simulink library "csu_rng_range_model_lib"  (R2015b)
settings: Solver=ode45  SolverMode=SingleTasking  StartTime=0.0  StopTime=10.0  RelTol=1e-3
values from neighbouring files (symbols this model uses):
  ldr_null_meas = -100    [csc_ldr_flir_lidar_init.m]
  ldr_use_meme_flag = 0    [csc_ldr_flir_lidar_init.m]
undefined symbols (not defined in the file or in its folder): ini_tgt_landing_mcmf_pos, ldr_100m_percent_error, ldr_100m_range_max, ldr_100m_range_min, ldr_2k_percent_error, ldr_2k_range_max, ldr_2k_range_min, ldr_lander_dcm, ldr_position_in_lander, ldr_rate_counter
libraries: util_quat_lib x9, simulink x6, util_common_lib x6, util_info_lib x3, util_frame_rotation_lib x2, util_geodesy_lib x2
settings Model: Creator=eleanor  LastModifiedBy=Mark Agbayani
settings DataIOCC: SaveFormat=Array  SignalLoggingSaveFormat=ModelDataLogs
settings OptimizationCC: BlockReduction=off  BooleanDataType=off  ExpressionDepthLimit=2147483647
settings DebuggingCC: SaveWithParameterizedLinksMsg=none  UnderspecifiedInitializationDetection=Classic  MergeDetectMultiDrivingBlocksExec=none  SignalResolutionControl=TryResolveAllWithWarning  FcnCallInpInsideContextMsg=EnableAllAsWarning  StateNameClashWarn=warning  StrictBusMsg=Warning
settings HardwareCC: ProdBitPerPointer=32  ProdLargestAtomicFloat=None  ProdIntDivRoundTo=Undefined  ProdEndianess=Unspecified  ProdWordSize=32  ProdHWDeviceType=32-bit Generic  TargetUnknown=on
settings GRTTargetCC: GeneratePreprocessorConditionals=Disable all  CombineOutputUpdateFcns=off  GRTInterface=on
settings ConfigComp: CovModelRefEnable=Off  CovSFcnEnable=off

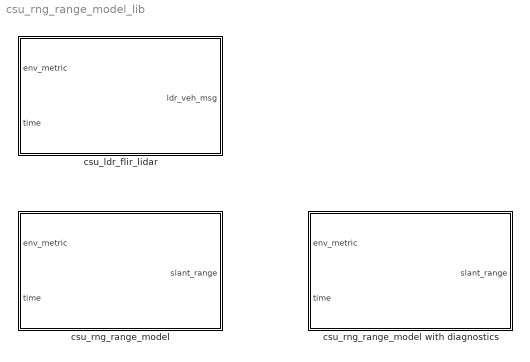
== system csu_rng_range_model_lib ==
  csu_ldr_flir_lidar : Subsystem  SystemSampleTime=0.1
  csu_rng_range_model : Subsystem  SystemSampleTime=0.1  mask{position_in_lander=ldr_position_in_lander, lander_dcm=ldr_lander_dcm}
      mask prompts: position_in_lander "LIDAR Position in Body Frame (meters)"; lander_dcm "LIDAR Attitude wrt Body Frame (DCM)"
  csu_rng_range_model with diagnostics : Subsystem  AncestorBlock=csu_rng_range_model_lib/csu_rng_range_model  SystemSampleTime=0.1  mask{position_in_lander=ldr_position_in_lander, lander_dcm=ldr_lander_dcm}
      mask prompts: position_in_lander "LIDAR Position in Body Frame (meters)"; lander_dcm "LIDAR Attitude wrt Body Frame (DCM)"

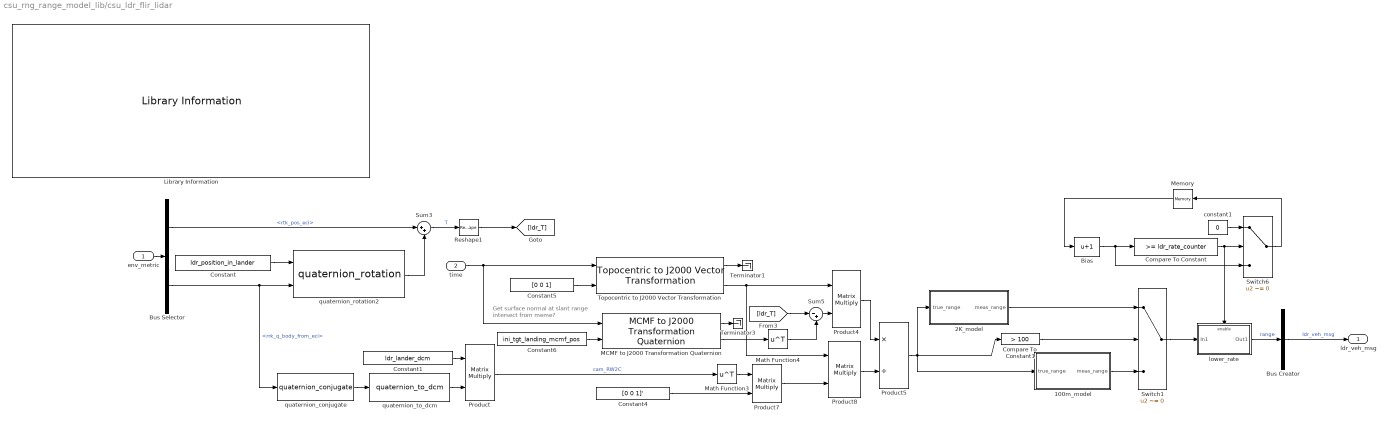
== system csu_rng_range_model_lib/csu_ldr_flir_lidar ==
  note: Get surface normal at slant range
      | intersect from meme?
  env_metric : Inport
  time : Inport  Port=2
  100m_model : Subsystem  TreatAsAtomicUnit=on
  2K_model : Subsystem  TreatAsAtomicUnit=on
  Bias : Bias  Bias=1
  Bus Creator : BusCreator  Inputs=1  OutDataTypeStr=Bus: ldr_veh_msg  NonVirtualBus=on
  Bus Selector : BusSelector  OutputSignals=lander_state_bus.rtk_pos_eci,lander_state_bus.rrk_q_body_from_eci
  Compare To Constant : simulink/Logic and Bit Operations/Compare To Constant  relop=>=  const=ldr_rate_counter  OutDataTypeStr=uint8
  Compare To Constant1 : simulink/Logic and Bit Operations/Compare To Constant  relop=>  const=100  OutDataTypeStr=uint8
  Constant : Constant  Value=ldr_position_in_lander
  Constant1 : Constant  Value=ldr_lander_dcm
  Constant4 : Constant  Value=[0 0 1]'  VectorParams1D=off
  Constant5 : Constant  Value=[0 0 1]  VectorParams1D=off
  Constant6 : Constant  Value=ini_tgt_landing_mcmf_pos  VectorParams1D=off
  Library Information : util_info_lib/Library Information  owner='NONE'
  MCMF to J2000 Transformation Quaternion : util_frame_rotation_lib/MCMF to J2000  Transformation Quaternion
  Math Function3 : Math  Operator=transpose  SaturateOnIntegerOverflow=on
  Math Function4 : Math  Operator=transpose  SaturateOnIntegerOverflow=on
  Memory : Memory  X0=ldr_rate_counter-1  InheritSampleTime=on
  Product{,4,7..8} (4 alike) : Product  Multiplication=Matrix(*)  RndMeth=Zero
  Product5 : Product  Inputs=*/  RndMeth=Zero
  Reshape1 : Reshape  OutputDimensionality=Column vector (2-D)
  Sum3 : Sum  Inputs=|++
  Sum5 : Sum  Inputs=|-+
  Switch1 : Switch  Criteria=u2 ~= 0  InputSameDT=on
  Switch6 : Switch  Criteria=u2 ~= 0  InputSameDT=on
  Terminator1 : Terminator
  Terminator3 : Terminator
  "Topocentric to J2000 Vector Transformation " : util_frame_rotation_lib/Topocentric to J2000 Vector Transformation   SystemSampleTime=-1
  constant1 : Constant  Value=0
  lower_rate : Subsystem  TreatAsAtomicUnit=on
  quaternion_conjugate : util_quat_lib/quaternion_conjugate  SystemSampleTime=-1
  quaternion_rotation2 : util_quat_lib/quaternion_rotation  SystemSampleTime=-1
  quaternion_to_dcm : util_quat_lib/quaternion_to_dcm  SystemSampleTime=-1
  ldr_veh_msg : Outport
  wires:
  quaternion_conjugate/1 -> quaternion_to_dcm/1
  2K_model/1(meas_range) -> Switch1/1
  100m_model/1(meas_range) -> Switch1/3
  Compare To Constant1/1 -> Switch1/2
  Product5/1 -> Compare To Constant1/1, 2K_model/1(true_range), 100m_model/1(true_range)
  Constant4/1 -> Product7/2
  "Topocentric to J2000 Vector Transformation "/1 -> Terminator1/1
  "Topocentric to J2000 Vector Transformation "/2 -> Product8/1, Product4/1
  time/1 -> MCMF to J2000 Transformation Quaternion/1, "Topocentric to J2000 Vector Transformation "/1
  Constant6/1 -> MCMF to J2000 Transformation Quaternion/2
  Constant5/1 -> "Topocentric to J2000 Vector Transformation "/2
  Constant/1 -> quaternion_rotation2/1
  quaternion_rotation2/1 -> Sum3/2
  Constant1/1 -> Product/1
  quaternion_to_dcm/1 -> Product/2
  Math Function4/1 -> Sum5/2
  MCMF to J2000 Transformation Quaternion/1 -> Terminator3/1
  MCMF to J2000 Transformation Quaternion/2 -> Math Function4/1
  Sum5/1 -> Product4/2
  [ldr_T] -> Sum5/1
  Math Function3/1 -> Product7/1
  Reshape1/1 -> [ldr_T]
  Product7/1 -> Product8/2
  env_metric/1 -> Bus Selector/1
  Bus Selector/1 -> Sum3/1  "<rtk_pos_eci>"
  Bus Selector/2 -> quaternion_conjugate/1, quaternion_rotation2/2  "<rrk_q_body_from_eci>"
  Product/1 -> Math Function3/1  "cam_RW2C"
  Sum3/1 -> Reshape1/1  "T"
  Product4/1 -> Product5/1
  Product8/1 -> Product5/2
  Memory/1 -> Bias/1
  Switch6/1 -> Memory/1
  Compare To Constant/1 -> lower_rate/Enable, Switch6/2
  Bias/1 -> Switch6/3, Compare To Constant/1
  constant1/1 -> Switch6/1
  lower_rate/1(Out1) -> Bus Creator/1  "range"
  Bus Creator/1 -> ldr_veh_msg/1  "ldr_veh_msg"
  Switch1/1 -> lower_rate/1(In1)

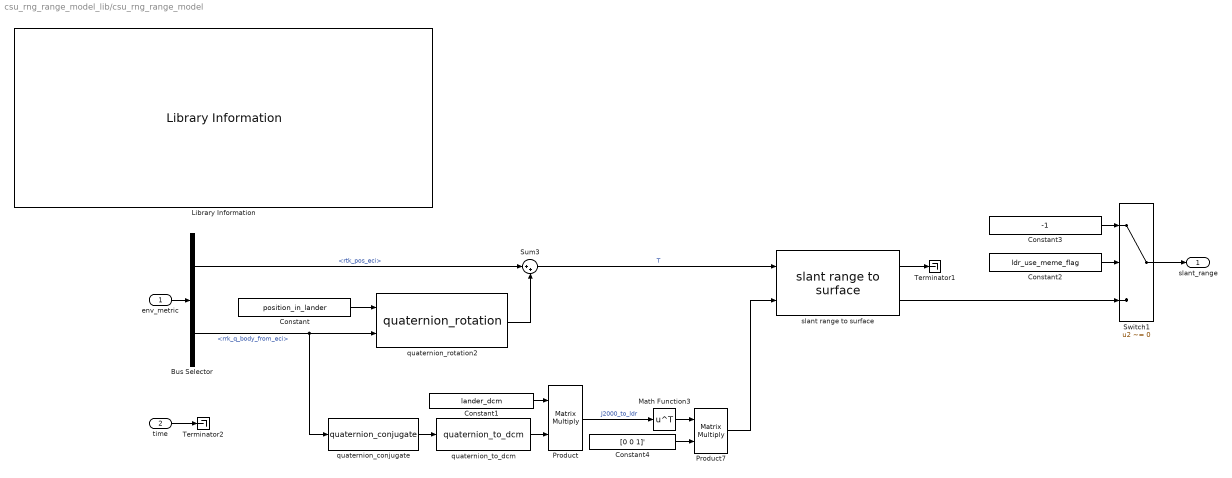
== system csu_rng_range_model_lib/csu_rng_range_model ==
  env_metric : Inport
  time : Inport  Port=2
  Bus Selector : BusSelector  OutputSignals=lander_state_bus.rtk_pos_eci,lander_state_bus.rrk_q_body_from_eci
  Constant : Constant  Value=position_in_lander
  Constant1 : Constant  Value=lander_dcm
  Constant2 : Constant  Value=ldr_use_meme_flag
  Constant3 : Constant  Value=-1
  Constant4 : Constant  Value=[0 0 1]'  VectorParams1D=off
  Library Information : util_info_lib/Library Information  owner='NONE'
  Math Function3 : Math  Operator=transpose  SaturateOnIntegerOverflow=on
  Product : Product  Multiplication=Matrix(*)  RndMeth=Zero
  Product7 : Product  Multiplication=Matrix(*)  RndMeth=Zero
  Sum3 : Sum  Inputs=|++
  Switch1 : Switch  Criteria=u2 ~= 0  InputSameDT=on
  Terminator1 : Terminator
  Terminator2 : Terminator
  quaternion_conjugate : util_quat_lib/quaternion_conjugate  SystemSampleTime=-1
  quaternion_rotation2 : util_quat_lib/quaternion_rotation  SystemSampleTime=-1
  quaternion_to_dcm : util_quat_lib/quaternion_to_dcm  SystemSampleTime=-1
  slant range to surface : util_geodesy_lib/slant range to surface
  slant_range : Outport
  wires:
  Product7/1 -> slant range to surface/2
  Sum3/1 -> slant range to surface/1  "T"
  quaternion_conjugate/1 -> quaternion_to_dcm/1
  Constant4/1 -> Product7/2
  Constant1/1 -> Product/1
  quaternion_to_dcm/1 -> Product/2
  Math Function3/1 -> Product7/1
  Product/1 -> Math Function3/1  "J2000_to_ldr"
  time/1 -> Terminator2/1
  slant range to surface/1 -> Terminator1/1
  Constant/1 -> quaternion_rotation2/1
  quaternion_rotation2/1 -> Sum3/2
  env_metric/1 -> Bus Selector/1
  Bus Selector/1 -> Sum3/1  "<rtk_pos_eci>"
  Bus Selector/2 -> quaternion_rotation2/2, quaternion_conjugate/1  "<rrk_q_body_from_eci>"
  Switch1/1 -> slant_range/1
  slant range to surface/2 -> Switch1/3
  Constant2/1 -> Switch1/2
  Constant3/1 -> Switch1/1

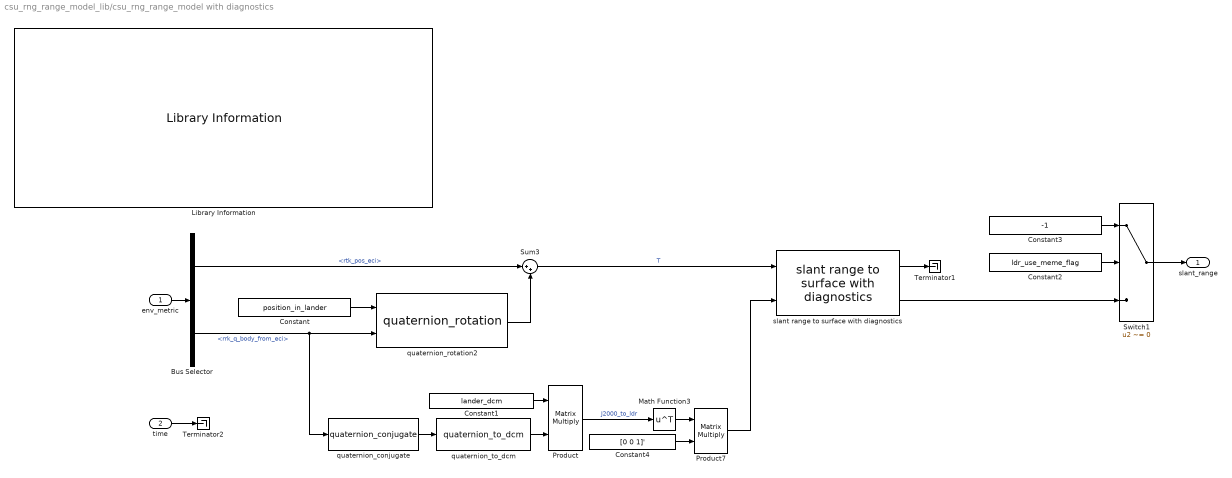
== system csu_rng_range_model_lib/csu_rng_range_model with diagnostics ==
  env_metric : Inport
  time : Inport  Port=2
  Bus Selector : BusSelector  OutputSignals=lander_state_bus.rtk_pos_eci,lander_state_bus.rrk_q_body_from_eci
  Constant : Constant  Value=position_in_lander
  Constant1 : Constant  Value=lander_dcm
  Constant2 : Constant  Value=ldr_use_meme_flag
  Constant3 : Constant  Value=-1
  Constant4 : Constant  Value=[0 0 1]'  VectorParams1D=off
  Library Information : util_info_lib/Library Information  owner='NONE'
  Math Function3 : Math  Operator=transpose  SaturateOnIntegerOverflow=on
  Product : Product  Multiplication=Matrix(*)  RndMeth=Zero
  Product7 : Product  Multiplication=Matrix(*)  RndMeth=Zero
  Sum3 : Sum  Inputs=|++
  Switch1 : Switch  Criteria=u2 ~= 0  InputSameDT=on
  Terminator1 : Terminator
  Terminator2 : Terminator
  quaternion_conjugate : util_quat_lib/quaternion_conjugate  SystemSampleTime=-1
  quaternion_rotation2 : util_quat_lib/quaternion_rotation  SystemSampleTime=-1
  quaternion_to_dcm : util_quat_lib/quaternion_to_dcm  SystemSampleTime=-1
  slant range to surface with diagnostics : util_geodesy_lib/slant range to surface with diagnostics
  slant_range : Outport
  wires:
  Constant3/1 -> Switch1/1
  Constant2/1 -> Switch1/2
  slant range to surface with diagnostics/2 -> Switch1/3
  Switch1/1 -> slant_range/1
  Bus Selector/2 -> quaternion_conjugate/1, quaternion_rotation2/2  "<rrk_q_body_from_eci>"
  Bus Selector/1 -> Sum3/1  "<rtk_pos_eci>"
  env_metric/1 -> Bus Selector/1
  quaternion_rotation2/1 -> Sum3/2
  Constant/1 -> quaternion_rotation2/1
  slant range to surface with diagnostics/1 -> Terminator1/1
  time/1 -> Terminator2/1
  Product/1 -> Math Function3/1  "J2000_to_ldr"
  Math Function3/1 -> Product7/1
  quaternion_to_dcm/1 -> Product/2
  Constant1/1 -> Product/1
  Constant4/1 -> Product7/2
  quaternion_conjugate/1 -> quaternion_to_dcm/1
  Sum3/1 -> slant range to surface with diagnostics/1  "T"
  Product7/1 -> slant range to surface with diagnostics/2

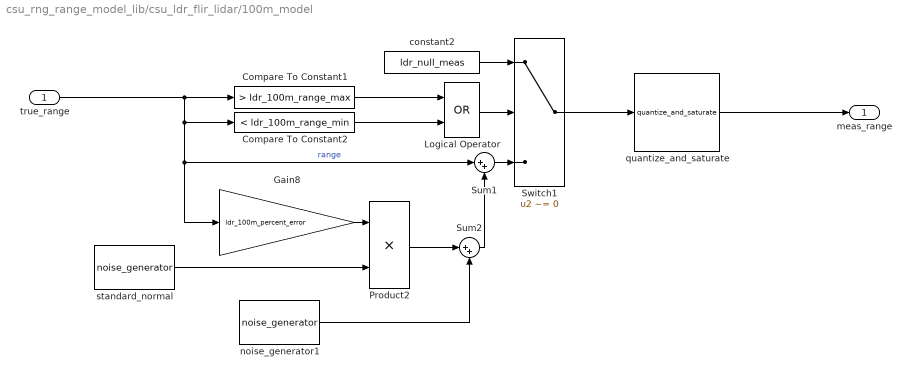
== system csu_rng_range_model_lib/csu_ldr_flir_lidar/100m_model ==
  true_range : Inport
  Compare To Constant1 : simulink/Logic and Bit Operations/Compare To Constant  relop=>  const=ldr_100m_range_max  OutDataTypeStr=uint8
  Compare To Constant2 : simulink/Logic and Bit Operations/Compare To Constant  relop=<  const=ldr_100m_range_min  OutDataTypeStr=uint8
  Gain8 : Gain  Gain=ldr_100m_percent_error
  Logical Operator : Logic  Operator=OR  AllPortsSameDT=off  OutDataTypeStr=boolean
  Product2 : Product  RndMeth=Zero
  Sum1 : Sum  Inputs=|++
  Sum2 : Sum  Inputs=|++
  Switch1 : Switch  Criteria=u2 ~= 0
  constant2 : Constant  Value=ldr_null_meas
  noise_generator1 : util_common_lib/noise_generator  std_dev=ldr_100m_1sig_noise  bias=0  seed=100  on=1  sample_time=sim_time_step_size
  quantize_and_saturate : util_common_lib/quantize_and_saturate  RES=ldr_100m_resolution  OPER=round  out_min=-inf  out_max=inf
  standard_normal : util_common_lib/noise_generator  std_dev=1  bias=0  seed=1  on=1  sample_time=sim_time_step_size
  meas_range : Outport
  wires:
  quantize_and_saturate/1 -> meas_range/1
  Switch1/1 -> quantize_and_saturate/1
  true_range/1 -> Compare To Constant1/1, Compare To Constant2/1, Gain8/1, Sum1/1  "range"
  Gain8/1 -> Product2/1
  standard_normal/1 -> Product2/2
  Product2/1 -> Sum2/1
  noise_generator1/1 -> Sum2/2
  Compare To Constant1/1 -> Logical Operator/1
  Compare To Constant2/1 -> Logical Operator/2
  Logical Operator/1 -> Switch1/2
  Sum1/1 -> Switch1/3
  Sum2/1 -> Sum1/2
  constant2/1 -> Switch1/1

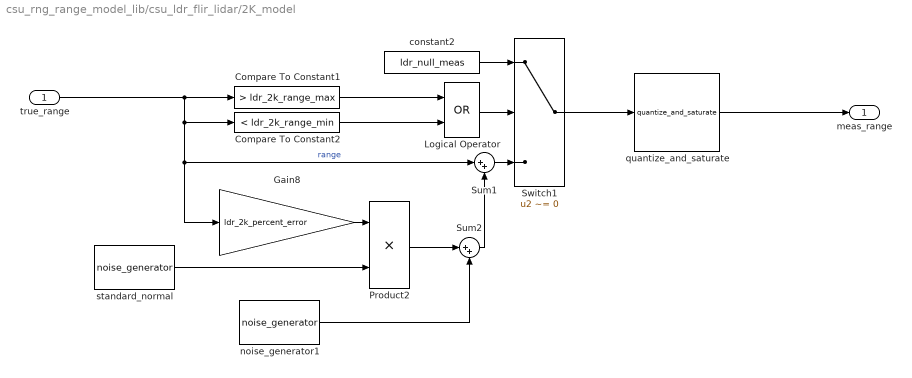
== system csu_rng_range_model_lib/csu_ldr_flir_lidar/2K_model ==
  true_range : Inport
  Compare To Constant1 : simulink/Logic and Bit Operations/Compare To Constant  relop=>  const=ldr_2k_range_max  OutDataTypeStr=uint8
  Compare To Constant2 : simulink/Logic and Bit Operations/Compare To Constant  relop=<  const=ldr_2k_range_min  OutDataTypeStr=uint8
  Gain8 : Gain  Gain=ldr_2k_percent_error
  Logical Operator : Logic  Operator=OR  AllPortsSameDT=off  OutDataTypeStr=boolean
  Product2 : Product  RndMeth=Zero
  Sum1 : Sum  Inputs=|++
  Sum2 : Sum  Inputs=|++
  Switch1 : Switch  Criteria=u2 ~= 0
  constant2 : Constant  Value=ldr_null_meas
  noise_generator1 : util_common_lib/noise_generator  std_dev=ldr_2k_1sig_noise  bias=0  seed=100  on=1  sample_time=sim_time_step_size
  quantize_and_saturate : util_common_lib/quantize_and_saturate  RES=ldr_2k_resolution  OPER=round  out_min=-inf  out_max=inf
  standard_normal : util_common_lib/noise_generator  std_dev=1  bias=0  seed=1  on=1  sample_time=sim_time_step_size
  meas_range : Outport
  wires:
  quantize_and_saturate/1 -> meas_range/1
  Switch1/1 -> quantize_and_saturate/1
  true_range/1 -> Compare To Constant1/1, Compare To Constant2/1, Gain8/1, Sum1/1  "range"
  Gain8/1 -> Product2/1
  standard_normal/1 -> Product2/2
  Product2/1 -> Sum2/1
  noise_generator1/1 -> Sum2/2
  Compare To Constant1/1 -> Logical Operator/1
  Compare To Constant2/1 -> Logical Operator/2
  Logical Operator/1 -> Switch1/2
  Sum1/1 -> Switch1/3
  Sum2/1 -> Sum1/2
  constant2/1 -> Switch1/1

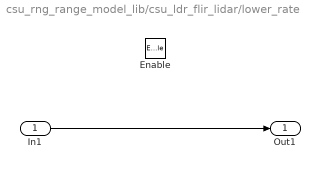
== system csu_rng_range_model_lib/csu_ldr_flir_lidar/lower_rate ==
  In1 : Inport
  Enable : EnablePort
  Out1 : Outport
  wires:
  In1/1 -> Out1/1
